simulink subsystem "Zona_muerta"  (R2024b)
settings: Solver=VariableStepAuto  StartTime=0.0  StopTime=10.0  RelTol=1e-3
settings Model: Creator=Ruben  LastModifiedBy=Ruben

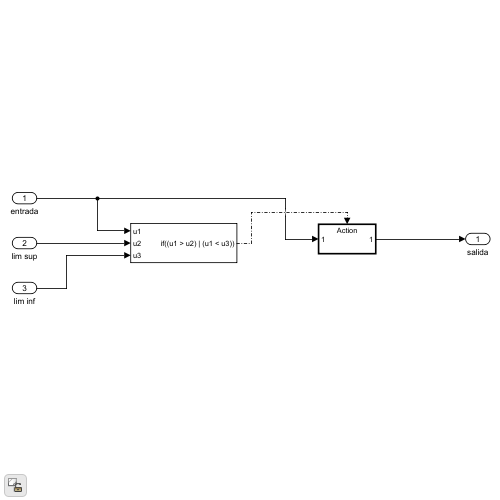
[thumbnail: Simulink's stored preview of the top-level diagram]
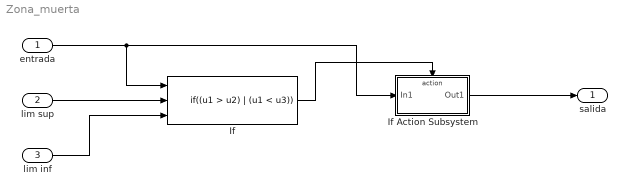
== system Zona_muerta ==
  entrada : Inport
  lim sup : Inport  Port=2
  lim inf : Inport  Port=3
  If : If  NumInputs=3  IfExpression=(u1 > u2) | (u1 < u3)  ShowElse=off
  If Action Subsystem : Subsystem  TreatAsAtomicUnit=on
  salida : Outport
  wires:
  entrada/1 -> If Action Subsystem/1(In1), If/1
  If Action Subsystem/1(Out1) -> salida/1
  If/1 -> If Action Subsystem/Action
  lim sup/1 -> If/2
  lim inf/1 -> If/3

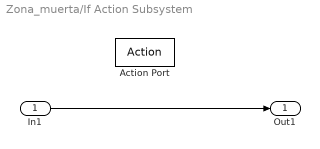
== system Zona_muerta/If Action Subsystem ==
  In1 : Inport
  Action Port : ActionPort
  Out1 : Outport  OutputWhenDisabled=reset  InitialOutput=0
  wires:
  In1/1 -> Out1/1
